simulink model "Open_loop"  (R2023b)
settings: Solver=VariableStepAuto  StartTime=0.0  StopTime=10.0  RelTol=1e-3
undefined symbols (not defined in the file): b_m, d_m, g, L_x_1, L_x_2, lx1, lx2, lx3, lx4, lx5, lx6, lx7, lx8, ly1, ly2, ly3, ly4, ly5, ly6, ly7, ly8, m
libraries: shared6dof x1
settings Model: Creator=Saif Mohamed  LastModifiedBy=Saif Mohamed

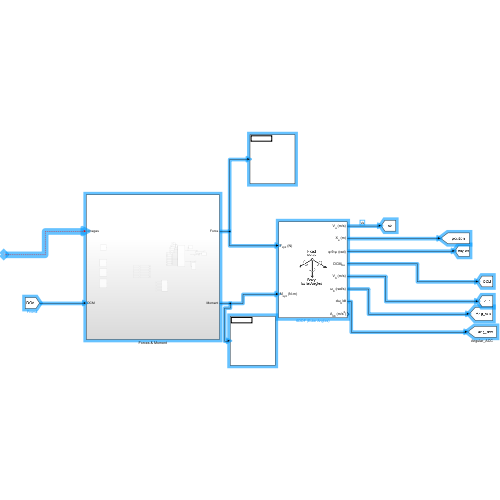
[thumbnail: Simulink's stored preview of the top-level diagram]
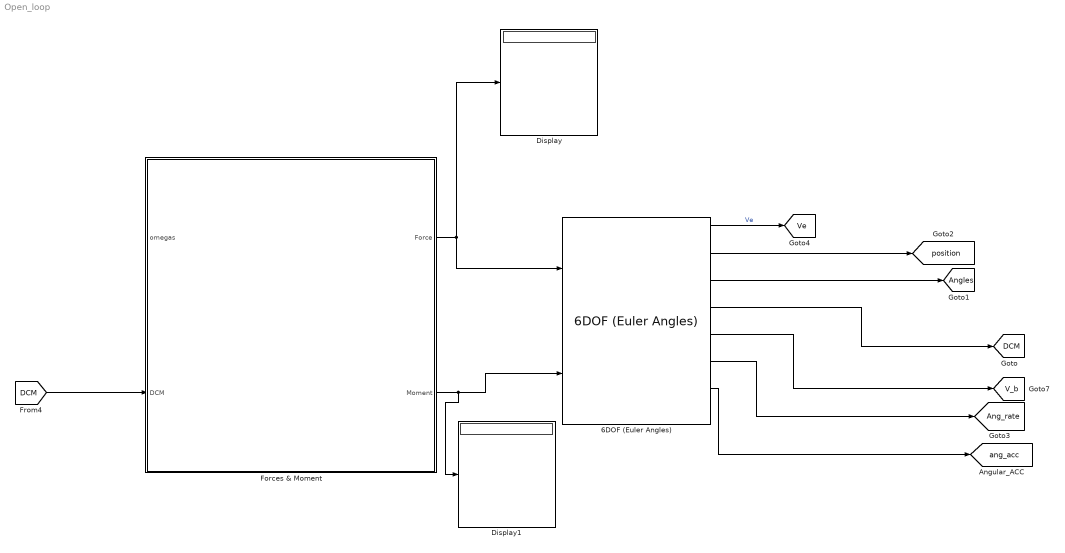
== system Open_loop ==
  6DOF (Euler Angles) : shared6dof/6DOF (Euler Angles)  units=Metric (MKS)  mtype=Fixed  rep=Euler Angles  xme_0=[0 0 0]  Vm_0=[0 0 0]  eul_0=[0 0 0]  pm_0=[0 0 0]  mass_0=m  mass_e=0.5  mass_f=2.0  inertia=I  inertia_e=eye(3)  inertia_f=2*eye(3)  k_quat=1.0  vre_flag=on  abi_flag=off  aMode=0  xme_statename=''  Vm_statename=''  eul_statename=''  quat_statename=''  pm_statename=''  mass_statename=''
  Display : Display
  Display1 : Display
  Forces & Moment : Subsystem
  tag scope: Ang_rate=global, Angles=global, DCM=global, V_b=global, Ve=global, ang_acc=global, position=global
  wires:
  Forces & Moment/2(Moment) -> Display1/1, 6DOF (Euler Angles)/2
  6DOF (Euler Angles)/7 -> [ang_acc]
  Forces & Moment/1(Force) -> 6DOF (Euler Angles)/1, Display/1
  6DOF (Euler Angles)/1 -> [Ve]  "Ve"
  6DOF (Euler Angles)/3 -> [Angles]
  6DOF (Euler Angles)/4 -> [DCM]
  6DOF (Euler Angles)/5 -> [V_b]
  6DOF (Euler Angles)/6 -> [Ang_rate]
  [DCM] -> Forces & Moment/2(DCM)
  6DOF (Euler Angles)/2 -> [position]
  ? -> Forces & Moment/1(omegas)

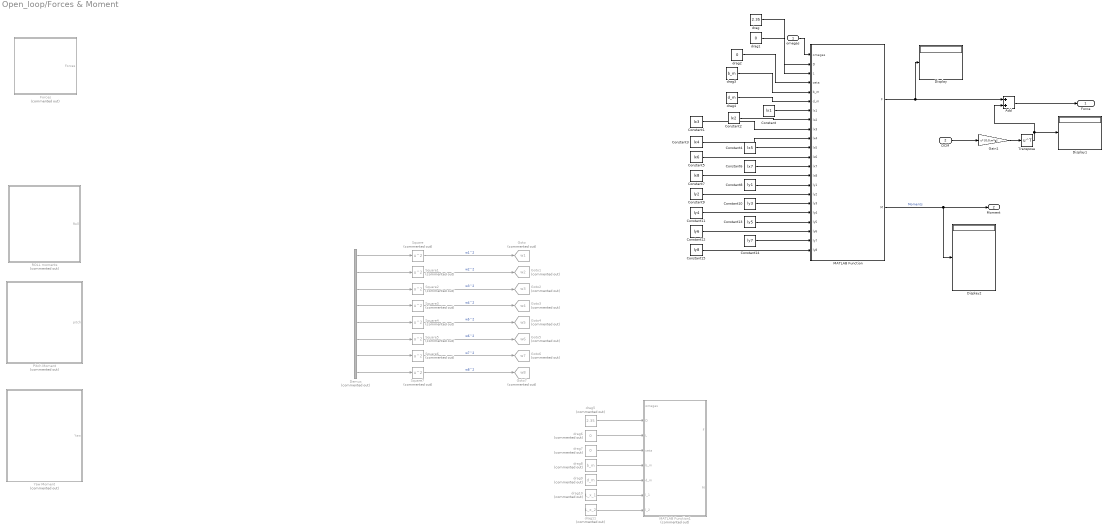
== system Open_loop/Forces & Moment ==
  omegas : Inport
  DCM : Inport  Port=2
  Add : Sum
  Constant : Constant  Value=lx1
  Constant1 : Constant  Value=lx3
  Constant10 : Constant  Value=ly3
  Constant11 : Constant  Value=ly4
  Constant12 : Constant  Value=ly6
  Constant13 : Constant  Value=ly5
  Constant14 : Constant  Value=ly7
  Constant15 : Constant  Value=ly8
  Constant2 : Constant  Value=lx2
  Constant3 : Constant  Value=lx4
  Constant4 : Constant  Value=lx5
  Constant5 : Constant  Value=lx6
  Constant6 : Constant  Value=lx7
  Constant7 : Constant  Value=lx8
  Constant8 : Constant  Value=ly1
  Constant9 : Constant  Value=ly2
  Demux : Demux  Commented=on  Outputs=8
  Display : Display
  Display1 : Display
  Display2 : Display
  Forces : Subsystem  Commented=on
  Gain1 : Gain  Gain=[0;0;m*g]  Multiplication=Matrix(u*K)
  Goto : Goto  Commented=on  GotoTag=w1  TagVisibility=global
  Goto1 : Goto  Commented=on  GotoTag=w2  TagVisibility=global
  Goto2 : Goto  Commented=on  GotoTag=w3  TagVisibility=global
  Goto3 : Goto  Commented=on  GotoTag=w4  TagVisibility=global
  Goto4 : Goto  Commented=on  GotoTag=w5  TagVisibility=global
  Goto5 : Goto  Commented=on  GotoTag=w6  TagVisibility=global
  Goto6 : Goto  Commented=on  GotoTag=w7  TagVisibility=global
  Goto7 : Goto  Commented=on  GotoTag=w8  TagVisibility=global
  MATLAB Function : MATLAB Function  TreatAsAtomicUnit=on
  MATLAB Function1 : MATLAB Function  Commented=on  TreatAsAtomicUnit=on
  Pitch Moment : Subsystem  Commented=on
  ROLL moments : Subsystem  Commented=on
  Square{,1..7} (8 alike) : Math  Commented=on  Operator=square
  Transpose : Math  Operator=transpose
  Yaw Moment : Subsystem  Commented=on
  drag : Constant  Value=2.35
  drag1 : Constant  Value=0
  drag10 : Constant  Commented=on  Value=L_x_1
  drag11 : Constant  Commented=on  Value=L_x_2
  drag2 : Constant  Value=0
  drag3 : Constant  Value=b_m
  drag4 : Constant  Value=d_m
  drag5 : Constant  Commented=on  Value=2.35
  drag6 : Constant  Commented=on  Value=0
  drag7 : Constant  Commented=on  Value=0
  drag8 : Constant  Commented=on  Value=b_m
  drag9 : Constant  Commented=on  Value=d_m
  Force : Outport
  Moment : Outport  Port=2
  wires:
  Square/1 -> Goto/1  "w1^2"
  Square1/1 -> Goto1/1  "w2^2"
  Square2/1 -> Goto2/1  "w3^2"
  Square3/1 -> Goto3/1  "w4^2"
  Square4/1 -> Goto4/1  "w5^2"
  Square5/1 -> Goto5/1  "w6^2"
  Square6/1 -> Goto6/1  "w7^2"
  Square7/1 -> Goto7/1  "w8^2"
  Demux/1 -> Square/1
  Demux/2 -> Square1/1
  Demux/3 -> Square2/1
  Demux/4 -> Square3/1
  Demux/5 -> Square4/1
  Demux/6 -> Square5/1
  Demux/7 -> Square6/1
  Demux/8 -> Square7/1
  Constant15/1 -> MATLAB Function/22(ly8)
  Constant2/1 -> MATLAB Function/8(lx2)
  Constant11/1 -> MATLAB Function/18(ly4)
  drag4/1 -> MATLAB Function/6(d_m)
  Gain1/1 -> Transpose/1
  Constant12/1 -> MATLAB Function/20(ly6)
  Constant9/1 -> MATLAB Function/16(ly2)
  Constant13/1 -> MATLAB Function/19(ly5)
  Constant10/1 -> MATLAB Function/17(ly3)
  Constant/1 -> MATLAB Function/7(lx1)
  Constant3/1 -> MATLAB Function/10(lx4)
  drag3/1 -> MATLAB Function/5(b_m)
  Constant1/1 -> MATLAB Function/9(lx3)
  Constant5/1 -> MATLAB Function/12(lx6)
  Constant8/1 -> MATLAB Function/15(ly1)
  DCM/1 -> Gain1/1
  drag1/1 -> MATLAB Function/3(L)
  Constant14/1 -> MATLAB Function/21(ly7)
  drag2/1 -> MATLAB Function/4(ceta)
  Transpose/1 -> Add/2, Display1/1
  Add/1 -> Force/1
  Constant4/1 -> MATLAB Function/11(lx5)
  Constant6/1 -> MATLAB Function/13(lx7)
  Constant7/1 -> MATLAB Function/14(lx8)
  drag/1 -> MATLAB Function/2(D)
  drag11/1 -> MATLAB Function1/8(l_2)
  drag8/1 -> MATLAB Function1/5(b_m)
  drag6/1 -> MATLAB Function1/3(L)
  drag5/1 -> MATLAB Function1/2(D)
  drag9/1 -> MATLAB Function1/6(d_m)
  drag10/1 -> MATLAB Function1/7(l_1)
  drag7/1 -> MATLAB Function1/4(ceta)
  omegas/1 -> MATLAB Function/1(omegas)
  MATLAB Function/1(F) -> Display/1, Add/1
  MATLAB Function/2(M) -> Moment/1, Display2/1  "Moments"

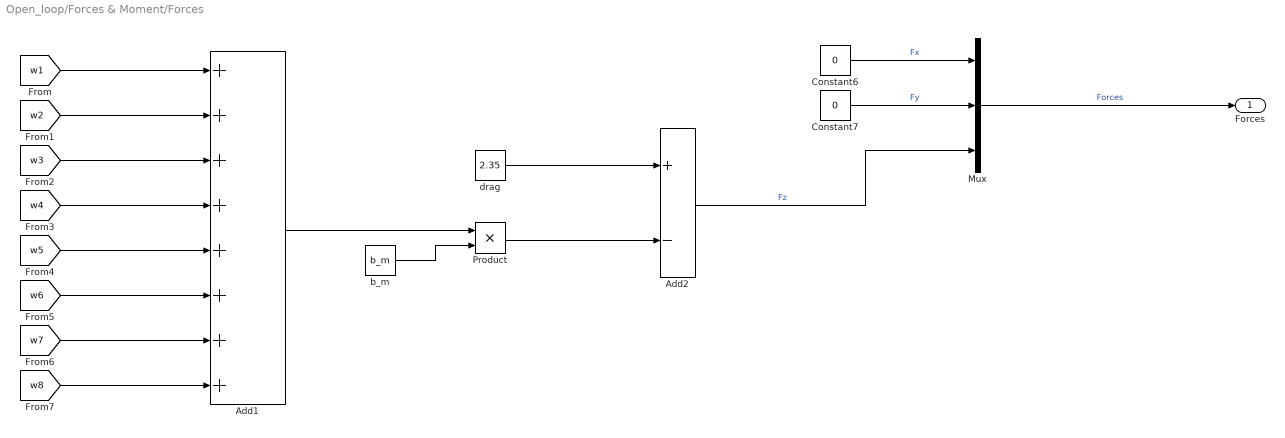
== system Open_loop/Forces & Moment/Forces ==
  Add1 : Sum  Inputs=++++++++
  Add2 : Sum  Inputs=+-
  Constant6 : Constant  Value=0
  Constant7 : Constant  Value=0
  Mux : Mux  Inputs=3
  Product : Product
  b_m : Constant  Value=b_m
  drag : Constant  Value=2.35
  Forces : Outport
  wires:
  Constant6/1 -> Mux/1  "Fx"
  [w4] -> Add1/4
  b_m/1 -> Product/2
  Product/1 -> Add2/2
  [w8] -> Add1/8
  drag/1 -> Add2/1
  Add1/1 -> Product/1
  Constant7/1 -> Mux/2  "Fy"
  [w7] -> Add1/7
  [w2] -> Add1/2
  [w1] -> Add1/1
  [w6] -> Add1/6
  [w3] -> Add1/3
  [w5] -> Add1/5
  Add2/1 -> Mux/3  "Fz"
  Mux/1 -> Forces/1  "Forces"

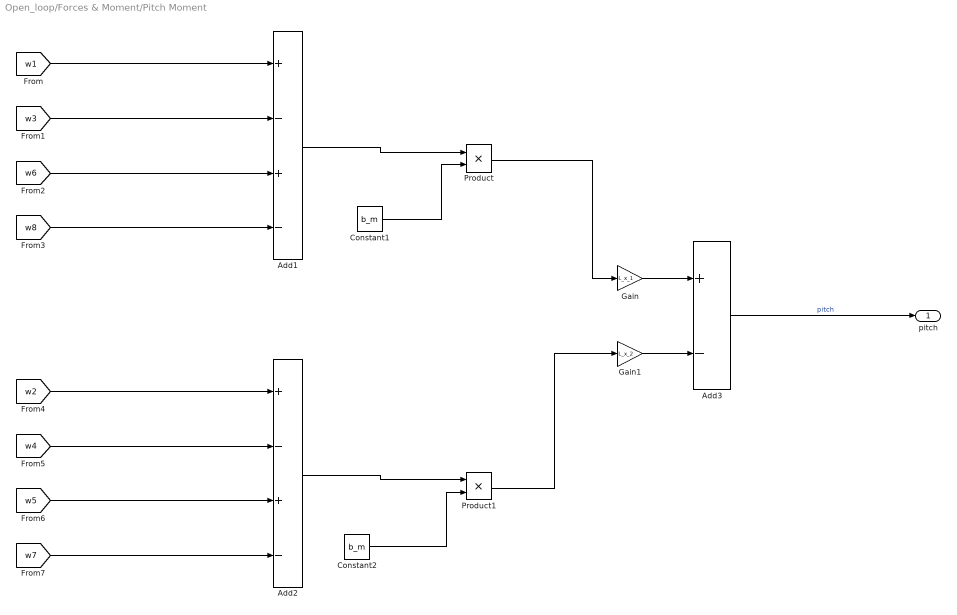
== system Open_loop/Forces & Moment/Pitch Moment ==
  Add1 : Sum  Inputs=+-+-
  Add2 : Sum  Inputs=+-+-
  Add3 : Sum  Inputs=+-
  Constant1 : Constant  Value=b_m
  Constant2 : Constant  Value=b_m
  Gain : Gain  Gain=L_x_1
  Gain1 : Gain  Gain=L_x_2
  Product : Product
  Product1 : Product
  pitch : Outport
  wires:
  Add1/1 -> Product/1
  [w3] -> Add1/2
  Add3/1 -> pitch/1  "pitch"
  [w7] -> Add2/4
  [w5] -> Add2/3
  [w4] -> Add2/2
  Add2/1 -> Product1/1
  [w2] -> Add2/1
  [w1] -> Add1/1
  [w6] -> Add1/3
  [w8] -> Add1/4
  Product1/1 -> Gain1/1
  Product/1 -> Gain/1
  Constant1/1 -> Product/2
  Constant2/1 -> Product1/2
  Gain/1 -> Add3/1
  Gain1/1 -> Add3/2

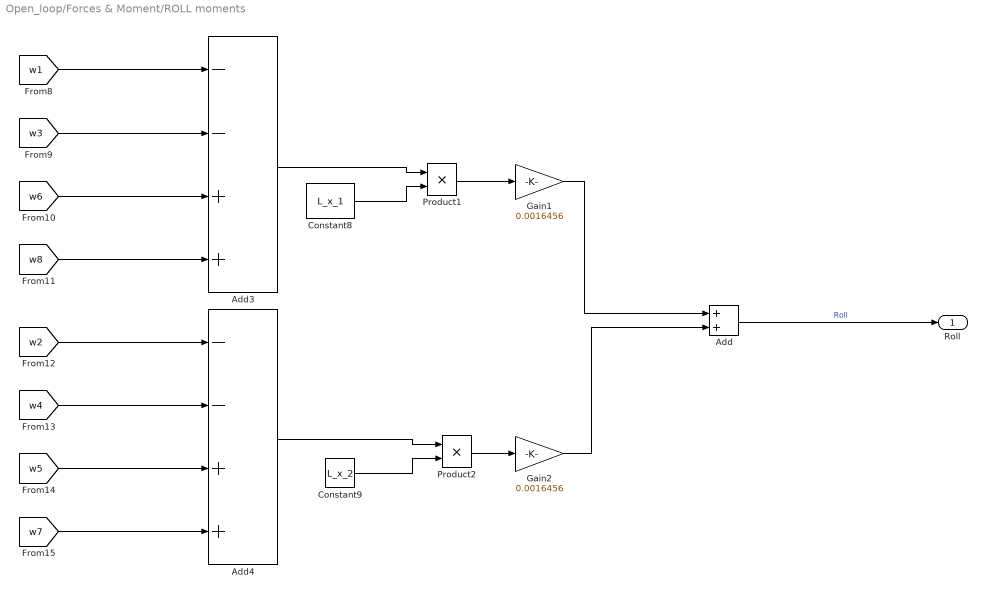
== system Open_loop/Forces & Moment/ROLL moments ==
  Add : Sum
  Add3 : Sum  Inputs=--++
  Add4 : Sum  Inputs=--++
  Constant8 : Constant  Value=L_x_1
  Constant9 : Constant  Value=L_x_2
  Gain1 : Gain  Gain=0.0016456
  Gain2 : Gain  Gain=0.0016456
  Product1 : Product
  Product2 : Product
  Roll : Outport
  wires:
  [w5] -> Add4/3
  [w2] -> Add4/1
  [w7] -> Add4/4
  [w3] -> Add3/2
  Constant9/1 -> Product2/2
  [w1] -> Add3/1
  [w4] -> Add4/2
  [w8] -> Add3/4
  [w6] -> Add3/3
  Product1/1 -> Gain1/1
  Constant8/1 -> Product1/2
  Product2/1 -> Gain2/1
  Add/1 -> Roll/1  "Roll"
  Add3/1 -> Product1/1
  Add4/1 -> Product2/1
  Gain2/1 -> Add/2
  Gain1/1 -> Add/1

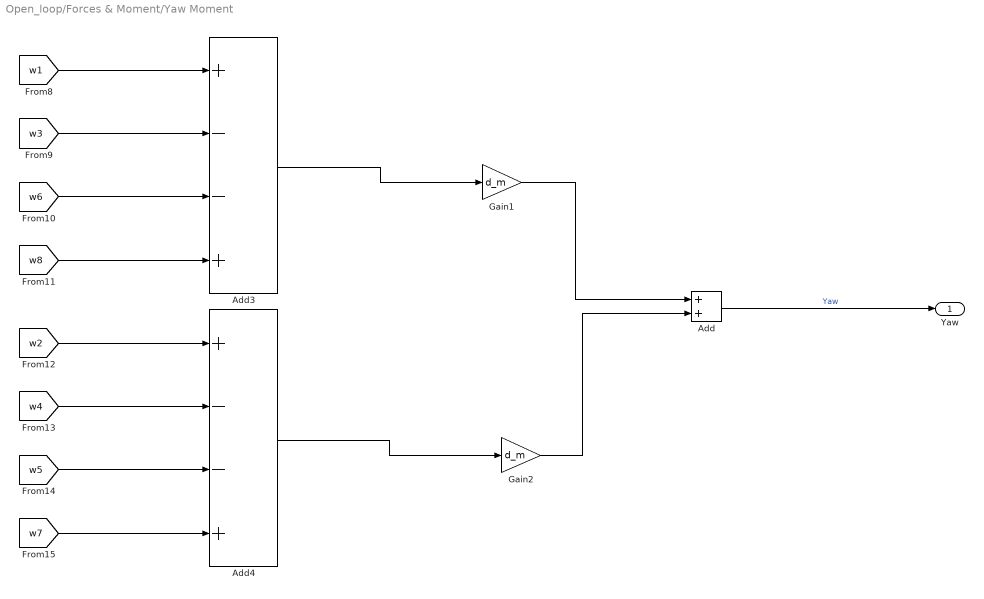
== system Open_loop/Forces & Moment/Yaw Moment ==
  Add : Sum
  Add3 : Sum  Inputs=+--+
  Add4 : Sum  Inputs=+--+
  Gain1 : Gain  Gain=d_m
  Gain2 : Gain  Gain=d_m
  Yaw : Outport
  wires:
  Add/1 -> Yaw/1  "Yaw"
  Add4/1 -> Gain2/1
  Add3/1 -> Gain1/1
  [w6] -> Add3/3
  [w8] -> Add3/4
  [w4] -> Add4/2
  [w1] -> Add3/1
  [w3] -> Add3/2
  [w7] -> Add4/4
  [w2] -> Add4/1
  [w5] -> Add4/3
  Gain2/1 -> Add/2
  Gain1/1 -> Add/1

== matlab function Open_loop/Forces & Moment/MATLAB Function ==
  data: omegas input size=[8,1]; D input; L input; ceta input; F output size=[1,3]; b_m input; d_m input; lx1 input; lx2 input; lx3 input; M output; lx4 input; lx5 input; lx6 input; lx7 input; lx8 input; ly1 input; ly2 input; ly3 input; ly4 input; ly5 input; ly6 input; ly7 input; ly8 input
function [F,M] = fcn(omegas,D,L,ceta, b_m,d_m,lx1,lx2, lx3, lx4, lx5, lx6, lx7, lx8, ly1, ly2, ly3, ly4, ly5, ly6, ly7, ly8)
w1=omegas(1);
w2=omegas(2);
w3=omegas(3);
w4=omegas(4);
w5=omegas(5);
w6=omegas(6);
w7=omegas(7);
w8=omegas(8);
F_F_z=b_m*(w1^2+w2^2+w6^2+w5^2)+b_m*(w8^2+w7^2+w4^2+w3^2);

Fx=0;
Fy=0;                            % Aerodynamic force needed 
Fz=D-F_F_z;                        % Aerodynamic force needed 
L_roll=(b_m*(-ly1*w1^2-ly4*w4^2-ly5*w5^2-ly8*w8^2))+(b_m)*(ly3*w3^2+ly2*w2^2+ly7*w7^2+ly6*w6^2);
M_Pitch=(b_m*(lx1*w1^2+lx3*w3^2+lx5*w5^2+lx7*w7^2))+(b_m*(-lx2*w2^2-lx4*w4^2-lx6*w6^2-lx8*w8^2));
N_yaw=d_m*((w1^2+w2^2+w5^2+w6^2)-(w3^2+w4^2+w7^2+w8^2));

F=[Fx Fy Fz];
M=[L_roll  M_Pitch N_yaw];

== matlab function Open_loop/Forces & Moment/MATLAB Function1 ==
  data: omegas input size=[8,1]; D input; L input; ceta input; F output size=[1,3]; b_m input; d_m input; l_1 input; l_2 input; M output
function [F,M] = fcn(omegas,D,L,ceta, b_m,d_m,l_1,l_2)
w1=omegas(1);
w2=omegas(2);
w3=omegas(3);
w4=omegas(4);
w5=omegas(5);
w6=omegas(6);
w7=omegas(7);
w8=omegas(8);
F_F_z=b_m*(w1^2+w2^2+w6^2+w5^2)+b_m*(w8^2+w7^2+w4^2+w3^2);

Fx=0;
Fy=0;                            % Aerodynamic force needed 
Fz=D-F_F_z;                        % Aerodynamic force needed 
L_roll=(b_m*l_1*(-w1^2-w3^2+w6^2+w8^2))+(b_m*l_2)*(-w2^2-w4^2+w7^2+w5^2);
M_Pitch=(b_m*l_1*(w1^2-w3^2+w6^2-w8^2))+(b_m*l_2*(w2^2-w4^2+w5^2-w7^2));
 N_yaw=(d_m*l_1*(w1^2-w3^2+w8^2-w6^2))+(d_m*l_2*(w2^2-w4^2+w7^2-w5^2));

F=[Fx Fy Fz];
M=[L_roll  M_Pitch N_yaw];
